simulink model "VB_RIFKF_GNSS_INS25"  (R2023a)
settings: Solver=FixedStepAuto  StartTime=0  StopTime=500  FixedStep=0.01  RelTol=1e-3
InitFcn:
  | resilient_initNavigation1216;
  | init_param;
undefined symbols (not defined in the file or in its folder): dt, g0, gam0_rad, ISUS_flag, magnitude, p, P0, P0_RIEKF, param, pd0, pe0, phi0_rad, pn0, psi, psi0_rad, state_dim, vd0, ve0, vn0
libraries: simulink_extras x68, dspstat3 x54, sharedtransform x47, simulink x43, matrix_library x9, sharedTrackingLibrary x5, dspfactors x4, aerolibconvert2 x3, aerolibtransform2 x3
(part 8 of 22)

== system VB_RIFKF_GNSS_INS25/ER EKF/Error State Kalman Filter/Extended Kalman Filter2 ==
  Q : Inport
  Enable1 : Inport  Port=2
  y1 : Inport  Port=3
  R1 : Inport  Port=4
  BlockOrdering : Constant  Value=true()  OutDataTypeStr=boolean
  Correct1 : Subsystem  AncestorBlock=sharedTrackingLibrary/Extras/EKFCorrect  TreatAsAtomicUnit=on  SystemSampleTime=p.SampleTimes.MeasurementFcn(1)  mask(EKFCorrect){ProcessedMaskData=p}
      mask init: same as VB_RIFKF_GNSS_INS25/ER EKF/Error State Kalman Filter/Extended Kalman Filter1/Correct1
      settings: LibrarySourceBlock=sharedTrackingLibrary/Extras/EKFCorrect
  DataStoreMemory - P : DataStoreMemory  DataStoreName=P  InitialValue=p.InitialCovariance  ShowAdditionalParam=off  OutDataTypeStr=p.DataType
  DataStoreMemory - x : DataStoreMemory  DataStoreName=x  InitialValue=p.InitialState  ShowAdditionalParam=off  OutDataTypeStr=p.DataType
  DataTypeConversion_Enable1 : DataTypeConversion  OutDataTypeStr=boolean  SaturateOnIntegerOverflow=off  RndMeth=Floor
  DataTypeConversion_Q : DataTypeConversion  OutDataTypeStr=p.DataType  SaturateOnIntegerOverflow=off  RndMeth=Floor
  DataTypeConversion_R1 : DataTypeConversion  OutDataTypeStr=p.DataType  SaturateOnIntegerOverflow=off  RndMeth=Floor
  DataTypeConversion_uMeas1 : DataTypeConversion  OutDataTypeStr=p.DataType  SaturateOnIntegerOverflow=off  RndMeth=Floor
  DataTypeConversion_uState : DataTypeConversion  OutDataTypeStr=p.DataType  SaturateOnIntegerOverflow=off  RndMeth=Floor
  DataTypeConversion_y1 : DataTypeConversion  OutDataTypeStr=p.DataType  SaturateOnIntegerOverflow=off  RndMeth=Floor
  MeasurementFcn1Inputs : Constant  Value=0  OutDataTypeStr=p.DataType  SampleTime=p.SampleTimes.MeasurementFcn(1)
  Output : Subsystem  TreatAsAtomicUnit=on  SystemSampleTime=p.SampleTimes.Output
  Predict : Subsystem  TreatAsAtomicUnit=on  SystemSampleTime=p.SampleTimes.StateTransitionFcn  mask(EKFPredict){ProcessedMaskData=p}
      mask init: same as VB_RIFKF_GNSS_INS25/ER EKF/Error State Kalman Filter/Extended Kalman Filter1/Predict
  StateTransitionFcnInputs : Constant  Value=0  OutDataTypeStr=p.DataType  SampleTime=p.SampleTimes.StateTransitionFcn
  checkMeasurementFcn1Signals : S-Function  FunctionName=ekfukfCheckSignals  Parameters=signalCheck.BlockPath, signalCheck.MeasurementFcn{1}.PortNames, signalCheck.MeasurementFcn{1}.SampleTime, signalCheck.DataType, signalCheck.MeasurementFcn{1}.PortDimensions, 1, signalCheck.MeasurementFcn{1}.HasAdditiveNoise  SFunctionDeploymentMode=off  EnableBusSupport=off
  checkStateTransitionFcnSignals : S-Function  FunctionName=ekfukfCheckSignals  Parameters=signalCheck.BlockPath, signalCheck.StateTransitionFcn.PortNames, signalCheck.StateTransitionFcn.SampleTime, signalCheck.DataType, signalCheck.StateTransitionFcn.PortDimensions, 0, signalCheck.StateTransitionFcn.HasAdditiveNoise  SFunctionDeploymentMode=off  EnableBusSupport=off
  xhat : Outport  VectorParamsAs1DForOutWhenUnconnected=off
  P : Outport  Port=2
  wires:
  y1/1 -> checkMeasurementFcn1Signals/2, DataTypeConversion_y1/1
  R1/1 -> checkMeasurementFcn1Signals/3, DataTypeConversion_R1/1
  Q/1 -> checkStateTransitionFcnSignals/1, DataTypeConversion_Q/1
  DataTypeConversion_Q/1 -> Predict/1(Q)
  Enable1/1 -> checkMeasurementFcn1Signals/1, DataTypeConversion_Enable1/1
  DataTypeConversion_Enable1/1 -> Correct1/Enable
  Output/2(P) -> P/1
  Output/1(x) -> xhat/1
  StateTransitionFcnInputs/1 -> checkStateTransitionFcnSignals/2, DataTypeConversion_uState/1
  DataTypeConversion_uState/1 -> Predict/2(uState)
  DataTypeConversion_y1/1 -> Correct1/1(yMeas)
  MeasurementFcn1Inputs/1 -> checkMeasurementFcn1Signals/4, DataTypeConversion_uMeas1/1
  DataTypeConversion_R1/1 -> Correct1/2(R)
  DataTypeConversion_uMeas1/1 -> Correct1/3(uMeas)
  BlockOrdering/1 -> [FirstOperation]
  [FirstOperation] -> Correct1/4(uBlockOrdering)
  [AfterCorrect] -> Output/1(uBlockOrdering)
  Output/3(yBlockOrdering) -> [AfterOutput]
  [AfterOutput] -> Predict/3(uBlockOrdering)
  Correct1/1(yBlockOrdering) -> [AfterCorrect]

== system VB_RIFKF_GNSS_INS25/ER EKF/Error State Kalman Filter/Simulink Function - GPS Measurements ==
  GPSMeasurementFcn : TriggerPort  TriggerType=function-call  IsSimulinkFunction=on  FunctionName=GPSMeasurementFcn  FunctionVisibility=scoped  VariantControl=Variant
  Add : Sum
  Constant6 : Constant  Value=[eye(6),zeros(6,9)]  OutDataTypeStr=single
  Product : Product  Multiplication=Matrix(*)
  x : ArgIn  DisableCoverage=on  OutDataTypeStr=single  PortDimensions=15  ArgumentName=x
  v : ArgIn  DisableCoverage=on  Port=2  OutDataTypeStr=single  PortDimensions=6  ArgumentName=v
  y : ArgOut  DisableCoverage=on  OutDataTypeStr=single  PortDimensions=6  ArgumentName=y
  wires:
  Add/1 -> y/1
  Product/1 -> Add/1
  x/1 -> Product/2
  Constant6/1 -> Product/1
  v/1 -> Add/2

== system VB_RIFKF_GNSS_INS25/ER EKF/Error State Kalman Filter/Simulink Function - GPS Measurements1 ==
  DCM_b_n : Inport
  DynamicMeasurementFcn_Dyn : TriggerPort  TriggerType=function-call  IsSimulinkFunction=on  FunctionName=DynamicMeasurementFcn_Dyn  FunctionVisibility=scoped  VariantControl=Variant
  Add : Sum  Commented=on
  Add1 : Sum
  Constant : Constant  Commented=on  Value=dt  OutDataTypeStr=single
  Constant6 : Constant  Value=[zeros(3,3),eye(3),zeros(3,12);zeros(3,15),eye(3)]  OutDataTypeStr=single
  Data Type Conversion6 : DataTypeConversion  Commented=on  OutDataTypeStr=single  SaturateOnIntegerOverflow=off  RndMeth=Floor
  From7 : From  Commented=on  GotoTag=DCM_b_n
  Goto : Goto  Commented=on  GotoTag=DCM_b_n
  MATLAB Function1 : MATLAB Function  Commented=on  TreatAsAtomicUnit=on
  Product : Product  Commented=on  Multiplication=Matrix(*)
  Product1 : Product  Multiplication=Matrix(*)
  x : ArgIn  DisableCoverage=on  OutDataTypeStr=single  PortDimensions=18  ArgumentName=x
  v : ArgIn  DisableCoverage=on  Port=2  OutDataTypeStr=single  PortDimensions=6  ArgumentName=v
  y : ArgOut  DisableCoverage=on  OutDataTypeStr=single  PortDimensions=6  ArgumentName=y
  wires:
  x/1 -> Product1/2
  Constant6/1 -> Product1/1
  Product1/1 -> Add1/1
  v/1 -> Add1/2
  Add1/1 -> y/1
  Data Type Conversion6/1 -> Product/1
  DCM_b_n/1 -> Goto/1
  Constant/1 -> MATLAB Function1/2(dt)
  From7/1 -> MATLAB Function1/1(Cbn)
  MATLAB Function1/1(H) -> Data Type Conversion6/1
  Product/1 -> Add/1

== system VB_RIFKF_GNSS_INS25/ER EKF/Error State Kalman Filter/Simulink Function - GPS Measurements2 ==
  ZUPTMeasurementFcn2 : TriggerPort  TriggerType=function-call  IsSimulinkFunction=on  FunctionName=ZUPTMeasurementFcn2  FunctionVisibility=scoped  VariantControl=Variant
  Add : Sum
  Constant6 : Constant  Value=[zeros(3,3),eye(3),zeros(3,12)]  OutDataTypeStr=single
  Product : Product  Multiplication=Matrix(*)
  x : ArgIn  DisableCoverage=on  OutDataTypeStr=single  PortDimensions=18  ArgumentName=x
  v : ArgIn  DisableCoverage=on  Port=2  OutDataTypeStr=single  PortDimensions=3  ArgumentName=v
  y : ArgOut  DisableCoverage=on  OutDataTypeStr=single  PortDimensions=3  ArgumentName=y
  wires:
  v/1 -> Add/2
  Constant6/1 -> Product/1
  x/1 -> Product/2
  Product/1 -> Add/1
  Add/1 -> y/1

== system VB_RIFKF_GNSS_INS25/ER EKF/Error State Kalman Filter/Simulink Function - State Transition ==
  DCM_b_n : Inport
  wxyz : Inport  Port=2
  fbxyz : Inport  Port=3
  stateTransitionFcn : TriggerPort  TriggerType=function-call  IsSimulinkFunction=on  FunctionName=stateTransitionFcn  FunctionVisibility=scoped  VariantControl=Variant
  Add : Sum
  Cal Phi : Subsystem
  Constant : Constant  Value=0.01  OutDataTypeStr=single
  Data Type Conversion1 : DataTypeConversion  OutDataTypeStr=single  SaturateOnIntegerOverflow=off  RndMeth=Floor
  Data Type Conversion6 : DataTypeConversion  OutDataTypeStr=single  SaturateOnIntegerOverflow=off  RndMeth=Floor
  MATLAB Function : MATLAB Function  TreatAsAtomicUnit=on
  Product1 : Product  Multiplication=Matrix(*)
  Product2 : Product  Multiplication=Matrix(*)
  Transpose : Math  Operator=transpose
  x : ArgIn  DisableCoverage=on  OutDataTypeStr=single  PortDimensions=15  ArgumentName=x
  w : ArgIn  Port=2  OutDataTypeStr=single  PortDimensions=12  ArgumentName=w
  xNext : ArgOut  DisableCoverage=on  OutDataTypeStr=single  PortDimensions=15  ArgumentName=xNext
  wires:
  Data Type Conversion6/1 -> Add/2
  Data Type Conversion1/1 -> Add/1
  Cal Phi/1(Phi) -> Product2/1
  fbxyz/1 -> [fbxyz]
  wxyz/1 -> [wxyz]
  DCM_b_n/1 -> [DCM_b_n]
  Constant/1 -> MATLAB Function/3(dt)
  [wxyz] -> MATLAB Function/2(wxyz)
  Transpose/1 -> MATLAB Function/1(Cnb)
  [DCM_b_n] -> Transpose/1
  [DCM_b_n] -> Cal Phi/1(<DCM_b_n>)
  [wxyz] -> Cal Phi/2(wxyz)
  [fbxyz] -> Cal Phi/3(axyz)
  Add/1 -> xNext/1
  Product1/1 -> Data Type Conversion1/1
  w/1 -> Product1/2
  MATLAB Function/1(G) -> Product1/1
  Product2/1 -> Data Type Conversion6/1
  x/1 -> Product2/2

== system VB_RIFKF_GNSS_INS25/ER EKF/Error State Kalman Filter/Simulink Function - State Transition Jacobian ==
  DCM_b_n : Inport
  wxyz : Inport  Port=2
  fbxyz : Inport  Port=3
  stateTransitionJacobianFcn : TriggerPort  TriggerType=function-call  IsSimulinkFunction=on  FunctionName=stateTransitionJacobianFcn  FunctionVisibility=scoped  VariantControl=Variant
  Cal Phi1 : Subsystem
  Constant : Constant  Value=0.01  OutDataTypeStr=single
  Data Type Conversion1 : DataTypeConversion  OutDataTypeStr=single  SaturateOnIntegerOverflow=off  RndMeth=Floor
  Data Type Conversion6 : DataTypeConversion  OutDataTypeStr=single  SaturateOnIntegerOverflow=off  RndMeth=Floor
  MATLAB Function : MATLAB Function  TreatAsAtomicUnit=on
  Terminator : Terminator
  Terminator1 : Terminator
  Transpose : Math  Operator=transpose
  x : ArgIn  DisableCoverage=on  OutDataTypeStr=single  PortDimensions=15  ArgumentName=x
  w : ArgIn  Port=2  OutDataTypeStr=single  PortDimensions=12  ArgumentName=w
  A : ArgOut  DisableCoverage=on  OutDataTypeStr=single  PortDimensions=[15 15]  ArgumentName=A
  G : ArgOut  Port=2  OutDataTypeStr=single  PortDimensions=[15 12]  ArgumentName=G
  wires:
  Data Type Conversion1/1 -> G/1
  Data Type Conversion6/1 -> A/1
  Constant/1 -> MATLAB Function/3(dt)
  Transpose/1 -> MATLAB Function/1(Cnb)
  [DCM_b_n] -> Transpose/1
  [wxyz] -> MATLAB Function/2(wxyz)
  [DCM_b_n] -> Cal Phi1/1(<DCM_b_n>)
  [fbxyz] -> Cal Phi1/3(axyz)
  [wxyz] -> Cal Phi1/2(wxyz)
  wxyz/1 -> [wxyz]
  fbxyz/1 -> [fbxyz]
  DCM_b_n/1 -> [DCM_b_n]
  Cal Phi1/1(Phi) -> Data Type Conversion6/1
  w/1 -> Terminator1/1
  x/1 -> Terminator/1
  MATLAB Function/1(G) -> Data Type Conversion1/1

== system VB_RIFKF_GNSS_INS25/ER EKF/Error State Kalman Filter/Subsystem ==
  data : Inport
  Detect Change : simulink/Logic and Bit Operations/Detect Change  vinit=0  InputProcessing=Columns as channels (frame based)  OutDataTypeStr=boolean
  Detect Change1 : simulink/Logic and Bit Operations/Detect Change  vinit=0  InputProcessing=Columns as channels (frame based)  OutDataTypeStr=boolean
  From Workspace2 : FromWorkspace  VariableName=[time(1:(end-1)),FCS1.data_hf_st.lat(1:(end-1))]
  From Workspace7 : FromWorkspace  Commented=on  VariableName=[All.t',All.vn]
  Selector : Selector  InputPortWidth=3  IndexOptions=Index vector (dialog)  Indices=[3]  OutputSizes=1
  Zero-Order Hold : ZeroOrderHold  SampleTime=0.2
  Zero-Order Hold1 : ZeroOrderHold  SampleTime=0.01
  flag : Outport
  wires:
  Zero-Order Hold/1 -> Selector/1
  data/1 -> Zero-Order Hold/1
  Selector/1 -> Zero-Order Hold1/1
  Detect Change1/1 -> flag/1
  Zero-Order Hold1/1 -> Detect Change/1
  From Workspace2/1 -> Detect Change1/1  "lat"

== system VB_RIFKF_GNSS_INS25/ER EKF/INS propogation/Init_PVQ ==
  QGC_sensor_reinit : Inport
  accl_B_m/s2_LPF : Inport  Port=2
  Magn_B_guess_LPF : Inport  Port=3
  pos_NED : Inport  Port=4
  vel_NED : Inport  Port=5
  Add : Sum
  Add1 : Sum
  Constant : Constant  Value=[0 0 0 1]  OutDataTypeStr=single
  Constant1 : Constant  OutDataTypeStr=uint8
  Constant2 : Constant  Value=[0;0;0]  OutDataTypeStr=single
  Constant3 : Constant  Value=[0;0;0]  OutDataTypeStr=single
  Constant4 : Constant  Value=[vn0;ve0;vd0]  OutDataTypeStr=single
  Constant5 : Constant  Value=[pn0;pe0;pd0]  OutDataTypeStr=single
  Detect Increase : simulink/Logic and Bit Operations/Detect Increase  vinit=0.0  OutDataTypeStr=boolean
  Horizontal_attitude : Subsystem  TreatAsAtomicUnit=on
  Horizontal_attitude2 : Subsystem  Commented=on  TreatAsAtomicUnit=on
  Memory : Memory
  Scope : Scope  NumInputPorts=2
  Scope1 : Scope
  Scope2 : Scope
  Subsystem : Subsystem
  Subsystem1 : Subsystem
  Switch{,1..3} (4 alike) : Switch  Criteria=u2 > Threshold  SaturateOnIntegerOverflow=off  InputSameDT=off
  quat_0 : Outport
  v0 : Outport  Port=2
  p0 : Outport  Port=3
  wires:
  Subsystem1/1(mean_data) -> Horizontal_attitude/2(Magn_mean_B_guess_LPF)
  Subsystem/1(mean_data) -> Horizontal_attitude/1(accl_mean_B_m/s_LPF)
  Memory/1 -> Switch1/3
  Constant/1 -> Switch/3
  Horizontal_attitude/1(quat_0) -> Switch/1
  Constant1/1 -> Switch1/1
  Switch1/1 -> Memory/1, Switch2/2, Switch3/2, Switch/2, Scope1/1
  accl_B_m/s2_LPF/1 -> Subsystem/1(data)
  QGC_sensor_reinit/1 -> Detect Increase/1, Scope/1
  Magn_B_guess_LPF/1 -> Subsystem1/1(data)
  Detect Increase/1 -> Horizontal_attitude/Enable, Switch1/2, Scope/2
  Constant2/1 -> Switch2/3
  Constant3/1 -> Switch3/3
  Switch2/1 -> v0/1
  Switch3/1 -> p0/1
  Add1/1 -> Switch3/1
  Switch/1 -> Scope2/1, quat_0/1
  Constant4/1 -> Add/2
  vel_NED/1 -> Add/1
  Add/1 -> Switch2/1
  pos_NED/1 -> Add1/1
  Constant5/1 -> Add1/2

== system VB_RIFKF_GNSS_INS25/ER EKF/INS propogation/accl bias compensation ==
  raw <accl_B_m/s2_LPF> : Inport
  dda : Inport  Port=2
  Add2 : Sum
  Data Type Conversion6 : DataTypeConversion  OutDataTypeStr=single  SaturateOnIntegerOverflow=off  RndMeth=Floor
  error compensation1 : Subsystem
  fb : Outport  PortDimensions=3
  da : Outport  Port=2  PortDimensions=3
  wires:
  error compensation1/1(da) -> da/1, Add2/2
  Add2/1 -> Data Type Conversion6/1
  Data Type Conversion6/1 -> fb/1
  raw <accl_B_m/s2_LPF>/1 -> Add2/1
  dda/1 -> error compensation1/1(dda)

== system VB_RIFKF_GNSS_INS25/ER EKF/INS propogation/att_update ==
  dtheta : Inport
  gyro : Inport  Port=2
  quat_0 : Inport  Port=3  PortDimensions=4
  init_flag : Inport  Port=4
  Bus Creator : BusCreator  Inputs=2
  Data Type Conversion1 : DataTypeConversion  OutDataTypeStr=single  SaturateOnIntegerOverflow=off  RndMeth=Floor
  Data Type Conversion2 : DataTypeConversion  OutDataTypeStr=single  SaturateOnIntegerOverflow=off  RndMeth=Floor
  Data Type Conversion3 : DataTypeConversion  OutDataTypeStr=double  SaturateOnIntegerOverflow=off  RndMeth=Floor
  Data Type Conversion4 : DataTypeConversion  OutDataTypeStr=double  SaturateOnIntegerOverflow=off  RndMeth=Floor
  Delay : Delay  DelayLength=1  InitialConditionSource=Input port  ExternalReset=Level hold
      settings: InputPortMap=u0,r5,p4
  Detect Increase : simulink/Logic and Bit Operations/Detect Increase  vinit=0.0  OutDataTypeStr=boolean
  Gain : Gain  Gain=dt  OutDataTypeStr=double
  Gain1 : Gain  Gain=-1
  JPLQuatMult : MATLAB Function  TreatAsAtomicUnit=on
  JPLQuatMult1 : MATLAB Function  TreatAsAtomicUnit=on
  JPLrv2q : MATLAB Function  TreatAsAtomicUnit=on
  JPLrv2q1 : MATLAB Function  TreatAsAtomicUnit=on
  MATLAB Function1 : MATLAB Function  TreatAsAtomicUnit=on
  Scope : Scope
  Transpose1 : Math  Operator=transpose  SignedPower=on
  att_update : Outport
  wires:
  JPLQuatMult/1(q_t) -> JPLQuatMult1/2(quatB)  "q_update"
  Detect Increase/1 -> Delay/2
  init_flag/1 -> Detect Increase/1
  Bus Creator/1 -> att_update/1
  Data Type Conversion2/1 -> Transpose1/1  "DCM_n_b"
  MATLAB Function1/1(Rot) -> Data Type Conversion2/1
  quat_0/1 -> Delay/3
  Delay/1 -> JPLQuatMult/2(quatB)
  Gain/1 -> JPLrv2q/1(rotVec)  "correctedDelAng"
  JPLrv2q/1(quaternion) -> JPLQuatMult/1(quatA)
  Data Type Conversion1/1 -> Bus Creator/1  "q_update"
  Data Type Conversion3/1 -> MATLAB Function1/1(q), Delay/1, Data Type Conversion1/1  "q_update"
  gyro/1 -> Gain/1
  Transpose1/1 -> Bus Creator/2  "DCM_b_n"
  Data Type Conversion4/1 -> JPLrv2q1/1(deltaTheta)  "q_update"
  JPLrv2q1/1(updateQuat) -> JPLQuatMult1/1(quatA)
  dtheta/1 -> Gain1/1
  Gain1/1 -> Scope/1, Data Type Conversion4/1
  JPLQuatMult1/1(q_t) -> Data Type Conversion3/1  "q_update"

== system VB_RIFKF_GNSS_INS25/ER EKF/INS propogation/gyro bias compensation ==
  raw <gyro_B_rad/s_LPF> : Inport
  ddg : Inport  Port=2
  Measuemrnt Enable Flag : Inport  Port=3
  Add1 : Sum
  Data Type Conversion4 : DataTypeConversion  OutDataTypeStr=single  SaturateOnIntegerOverflow=off  RndMeth=Floor
  Scope1 : Scope
  error compensation : Subsystem
  wb : Outport  PortDimensions=3
  dg : Outport  Port=2  PortDimensions=3
  wires:
  ddg/1 -> error compensation/1(ddg)
  Add1/1 -> Data Type Conversion4/1
  Measuemrnt Enable Flag/1 -> error compensation/2(Enable)
  error compensation/1(dg) -> dg/1, Scope1/1, Add1/2
  raw <gyro_B_rad/s_LPF>/1 -> Add1/1
  Data Type Conversion4/1 -> wb/1

== system VB_RIFKF_GNSS_INS25/ER EKF/INS propogation/vel_pos_update ==
  <DCM_b_n> : Inport
  Ab : Inport  Port=2
  v0 : Inport  Port=3
  p0 : Inport  Port=4
  QGC_init : Inport  Port=5
  dp : Inport  Port=6
  dv : Inport  Port=7
  Kinematic Equation : Subsystem
  QGC_init1 : InportShadow  Port=5
  pos update : Subsystem
  vel update : Subsystem
  p_k : Outport  PortDimensions=3
  V : Outport  Port=2  PortDimensions=3
  wires:
  <DCM_b_n>/1 -> Kinematic Equation/1(Cbn)
  Ab/1 -> Kinematic Equation/2(Ab)
  QGC_init/1 -> vel update/1(QGC_init)
  Kinematic Equation/1(An) -> vel update/2(An)
  dv/1 -> vel update/3(KFState_dv)
  v0/1 -> vel update/4(v0)
  dp/1 -> pos update/2(dp)
  p0/1 -> pos update/4(p0)
  pos update/1(p_k) -> p_k/1
  QGC_init1/1 -> pos update/3(QGC_init)
  vel update/1(vel_k) -> pos update/1(vel_k), V/1

== system VB_RIFKF_GNSS_INS25/ISUS_RIEKF1/Bus_Constructor2/Rotation_output ==
  RotationData : Inport
  Bus Creator : BusCreator  Inputs=4
  Bus Selector3 : BusSelector  OutputSignals=DCM_b_n
  Data Type Conversion1 : DataTypeConversion  OutDataTypeStr=single  SaturateOnIntegerOverflow=off  RndMeth=Floor
  Data Type Conversion11 : DataTypeConversion  OutDataTypeStr=single  SaturateOnIntegerOverflow=off  RndMeth=Floor
  Data Type Conversion12 : DataTypeConversion  OutDataTypeStr=double  SaturateOnIntegerOverflow=off  RndMeth=Floor
  Demux : Demux  Outputs=3
  Direction Cosine Matrix to Rotation Angles : sharedtransform/Direction Cosine Matrix to Rotation Angles  rotationOrder=ZYX  aMode=aMode  action=None  tolerance=eps(2)
      settings: LibrarySourceBlock=|
      | aerolibtransform2/Direction Cosine Matrix
      | to Rotation Angles
  Direction Cosine Matrix to Quaternions : sharedtransform/Direction Cosine Matrix  to Quaternions  aMode=0  action=None  tolerance=eps(2)
      settings: LibrarySourceBlock=|
      | aerolibtransform2/Direction Cosine Matrix
      | to Quaternions
  Radians to Degrees : simulink_extras/Transformations/Radians to Degrees
  Scope : Scope
  Signal Copy1 : SignalConversion  OverrideOpt=off
  Transpose : Math  Operator=transpose
  psi_theta_phi_rad : Outport
  wires:
  Direction Cosine Matrix to Quaternions/1 -> Data Type Conversion1/1  "q"
  Radians to Degrees/1 -> Data Type Conversion11/1
  Transpose/1 -> Data Type Conversion12/1
  Data Type Conversion12/1 -> Direction Cosine Matrix to Quaternions/1, Direction Cosine Matrix to Rotation Angles/1
  RotationData/1 -> Signal Copy1/1
  Signal Copy1/1 -> Bus Selector3/1
  Bus Selector3/1 -> Transpose/1  "<DCM_b_n>"
  Direction Cosine Matrix to Rotation Angles/1 -> Radians to Degrees/1
  Bus Creator/1 -> psi_theta_phi_rad/1
  Demux/1 -> Bus Creator/1  "psi_rad"
  Demux/2 -> Bus Creator/2  "theta_rad"
  Demux/3 -> Bus Creator/3, Scope/1  "phi_rad"
  Data Type Conversion11/1 -> Demux/1
  Data Type Conversion1/1 -> Bus Creator/4  "q"

== system VB_RIFKF_GNSS_INS25/ISUS_RIEKF1/Error State Kalman Filter M1/Cal Q1 ==
  Constant : Constant  Value=dt  OutDataTypeStr=double
  MATLAB Function1 : MATLAB Function  TreatAsAtomicUnit=on
  Qd : Outport
  wires:
  MATLAB Function1/1(Q) -> Qd/1
  Constant/1 -> MATLAB Function1/1(dt)

== system VB_RIFKF_GNSS_INS25/ISUS_RIEKF1/Error State Kalman Filter M1/Extended Kalman Filter M1 ==
  Q : Inport
  Enable1 : Inport  Port=2
  y1 : Inport  Port=3
  R1 : Inport  Port=4
  H : Inport  Port=5
  BlockOrdering : Constant  Value=true()  OutDataTypeStr=boolean
  Correct M1 : Subsystem  AncestorBlock=sharedTrackingLibrary/Extras/EKFCorrect  TreatAsAtomicUnit=on  SystemSampleTime=p.SampleTimes.MeasurementFcn(1)  mask(EKFCorrect){ProcessedMaskData=p}
      mask init: same as VB_RIFKF_GNSS_INS25/ER EKF/Error State Kalman Filter/Extended Kalman Filter1/Correct1
      settings: LibrarySourceBlock=sharedTrackingLibrary/Extras/EKFCorrect
  DataStoreMemory - P : DataStoreMemory  DataStoreName=P  InitialValue=p.InitialCovariance  ShowAdditionalParam=off  OutDataTypeStr=p.DataType
  DataStoreMemory - x : DataStoreMemory  DataStoreName=x  InitialValue=p.InitialState  ShowAdditionalParam=off  OutDataTypeStr=p.DataType
  DataTypeConversion_Enable1 : DataTypeConversion  OutDataTypeStr=boolean  SaturateOnIntegerOverflow=off  RndMeth=Floor
  DataTypeConversion_Q : DataTypeConversion  OutDataTypeStr=p.DataType  SaturateOnIntegerOverflow=off  RndMeth=Floor
  DataTypeConversion_R1 : DataTypeConversion  OutDataTypeStr=p.DataType  SaturateOnIntegerOverflow=off  RndMeth=Floor
  DataTypeConversion_uMeas1 : DataTypeConversion  OutDataTypeStr=p.DataType  SaturateOnIntegerOverflow=off  RndMeth=Floor
  DataTypeConversion_uState : DataTypeConversion  OutDataTypeStr=p.DataType  SaturateOnIntegerOverflow=off  RndMeth=Floor
  DataTypeConversion_y1 : DataTypeConversion  OutDataTypeStr=p.DataType  SaturateOnIntegerOverflow=off  RndMeth=Floor
  MeasurementFcn1Inputs : Constant  Value=0  OutDataTypeStr=p.DataType  SampleTime=p.SampleTimes.MeasurementFcn(1)
  Output : Subsystem  TreatAsAtomicUnit=on  SystemSampleTime=p.SampleTimes.Output
  Predict : Subsystem  TreatAsAtomicUnit=on  SystemSampleTime=p.SampleTimes.StateTransitionFcn  mask(EKFPredict){ProcessedMaskData=p}
      mask init: same as VB_RIFKF_GNSS_INS25/ER EKF/Error State Kalman Filter/Extended Kalman Filter1/Predict
  StateTransitionFcnInputs : Constant  Value=0  OutDataTypeStr=p.DataType  SampleTime=p.SampleTimes.StateTransitionFcn
  checkMeasurementFcn1Signals : S-Function  FunctionName=ekfukfCheckSignals  Parameters=signalCheck.BlockPath, signalCheck.MeasurementFcn{1}.PortNames, signalCheck.MeasurementFcn{1}.SampleTime, signalCheck.DataType, signalCheck.MeasurementFcn{1}.PortDimensions, 1, signalCheck.MeasurementFcn{1}.HasAdditiveNoise  SFunctionDeploymentMode=off  EnableBusSupport=off
  checkStateTransitionFcnSignals : S-Function  FunctionName=ekfukfCheckSignals  Parameters=signalCheck.BlockPath, signalCheck.StateTransitionFcn.PortNames, signalCheck.StateTransitionFcn.SampleTime, signalCheck.DataType, signalCheck.StateTransitionFcn.PortDimensions, 0, signalCheck.StateTransitionFcn.HasAdditiveNoise  SFunctionDeploymentMode=off  EnableBusSupport=off
  xhat : Outport  VectorParamsAs1DForOutWhenUnconnected=off
  P : Outport  Port=2
  wires:
  Output/2(P) -> P/1
  Correct M1/1(yBlockOrdering) -> [AfterCorrect]
  Output/1(x) -> xhat/1
  y1/1 -> checkMeasurementFcn1Signals/2, DataTypeConversion_y1/1
  R1/1 -> checkMeasurementFcn1Signals/3, DataTypeConversion_R1/1
  Q/1 -> checkStateTransitionFcnSignals/1, DataTypeConversion_Q/1
  DataTypeConversion_Q/1 -> Predict/1(Q)
  Enable1/1 -> checkMeasurementFcn1Signals/1, DataTypeConversion_Enable1/1
  DataTypeConversion_Enable1/1 -> Correct M1/Enable
  StateTransitionFcnInputs/1 -> checkStateTransitionFcnSignals/2, DataTypeConversion_uState/1
  DataTypeConversion_uState/1 -> Predict/2(uState)
  DataTypeConversion_y1/1 -> Correct M1/1(yMeas)
  MeasurementFcn1Inputs/1 -> checkMeasurementFcn1Signals/4, DataTypeConversion_uMeas1/1
  DataTypeConversion_R1/1 -> Correct M1/2(R)
  DataTypeConversion_uMeas1/1 -> Correct M1/3(uMeas)
  BlockOrdering/1 -> [FirstOperation]
  [FirstOperation] -> Correct M1/4(uBlockOrdering)
  [AfterCorrect] -> Output/1(uBlockOrdering)
  Output/3(yBlockOrdering) -> [AfterOutput]
  [AfterOutput] -> Predict/3(uBlockOrdering)
  H/1 -> Correct M1/5(H)

== system VB_RIFKF_GNSS_INS25/ISUS_RIEKF1/Error State Kalman Filter M1/Extended Kalman Filter M2 ==
  Q : Inport
  Enable1 : Inport  Port=2
  y1 : Inport  Port=3
  R1 : Inport  Port=4
  BlockOrdering : Constant  Value=true()  OutDataTypeStr=boolean
  Correct M1 : Subsystem  AncestorBlock=sharedTrackingLibrary/Extras/EKFCorrect  TreatAsAtomicUnit=on  SystemSampleTime=p.SampleTimes.MeasurementFcn(1)  mask(EKFCorrect){ProcessedMaskData=p}
      mask init: same as VB_RIFKF_GNSS_INS25/ER EKF/Error State Kalman Filter/Extended Kalman Filter1/Correct1
      settings: LibrarySourceBlock=sharedTrackingLibrary/Extras/EKFCorrect
  DataStoreMemory - P : DataStoreMemory  DataStoreName=P  InitialValue=p.InitialCovariance  ShowAdditionalParam=off  OutDataTypeStr=p.DataType
  DataStoreMemory - x : DataStoreMemory  DataStoreName=x  InitialValue=p.InitialState  ShowAdditionalParam=off  OutDataTypeStr=p.DataType
  DataTypeConversion_Enable1 : DataTypeConversion  OutDataTypeStr=boolean  SaturateOnIntegerOverflow=off  RndMeth=Floor
  DataTypeConversion_Q : DataTypeConversion  OutDataTypeStr=p.DataType  SaturateOnIntegerOverflow=off  RndMeth=Floor
  DataTypeConversion_R1 : DataTypeConversion  OutDataTypeStr=p.DataType  SaturateOnIntegerOverflow=off  RndMeth=Floor
  DataTypeConversion_uMeas1 : DataTypeConversion  OutDataTypeStr=p.DataType  SaturateOnIntegerOverflow=off  RndMeth=Floor
  DataTypeConversion_uState : DataTypeConversion  OutDataTypeStr=p.DataType  SaturateOnIntegerOverflow=off  RndMeth=Floor
  DataTypeConversion_y1 : DataTypeConversion  OutDataTypeStr=p.DataType  SaturateOnIntegerOverflow=off  RndMeth=Floor
  MeasurementFcn1Inputs : Constant  Value=0  OutDataTypeStr=p.DataType  SampleTime=p.SampleTimes.MeasurementFcn(1)
  Output : Subsystem  TreatAsAtomicUnit=on  SystemSampleTime=p.SampleTimes.Output
  Predict : Subsystem  TreatAsAtomicUnit=on  SystemSampleTime=p.SampleTimes.StateTransitionFcn  mask(EKFPredict){ProcessedMaskData=p}
      mask init: same as VB_RIFKF_GNSS_INS25/ER EKF/Error State Kalman Filter/Extended Kalman Filter1/Predict
  StateTransitionFcnInputs : Constant  Value=0  OutDataTypeStr=p.DataType  SampleTime=p.SampleTimes.StateTransitionFcn
  checkMeasurementFcn1Signals : S-Function  FunctionName=ekfukfCheckSignals  Parameters=signalCheck.BlockPath, signalCheck.MeasurementFcn{1}.PortNames, signalCheck.MeasurementFcn{1}.SampleTime, signalCheck.DataType, signalCheck.MeasurementFcn{1}.PortDimensions, 1, signalCheck.MeasurementFcn{1}.HasAdditiveNoise  SFunctionDeploymentMode=off  EnableBusSupport=off
  checkStateTransitionFcnSignals : S-Function  FunctionName=ekfukfCheckSignals  Parameters=signalCheck.BlockPath, signalCheck.StateTransitionFcn.PortNames, signalCheck.StateTransitionFcn.SampleTime, signalCheck.DataType, signalCheck.StateTransitionFcn.PortDimensions, 0, signalCheck.StateTransitionFcn.HasAdditiveNoise  SFunctionDeploymentMode=off  EnableBusSupport=off
  xhat : Outport  VectorParamsAs1DForOutWhenUnconnected=off
  P : Outport  Port=2
  wires:
  [AfterOutput] -> Predict/3(uBlockOrdering)
  Output/3(yBlockOrdering) -> [AfterOutput]
  [AfterCorrect] -> Output/1(uBlockOrdering)
  [FirstOperation] -> Correct M1/4(uBlockOrdering)
  BlockOrdering/1 -> [FirstOperation]
  DataTypeConversion_uMeas1/1 -> Correct M1/3(uMeas)
  DataTypeConversion_R1/1 -> Correct M1/2(R)
  MeasurementFcn1Inputs/1 -> DataTypeConversion_uMeas1/1, checkMeasurementFcn1Signals/4
  DataTypeConversion_y1/1 -> Correct M1/1(yMeas)
  DataTypeConversion_uState/1 -> Predict/2(uState)
  StateTransitionFcnInputs/1 -> DataTypeConversion_uState/1, checkStateTransitionFcnSignals/2
  DataTypeConversion_Enable1/1 -> Correct M1/Enable
  Enable1/1 -> DataTypeConversion_Enable1/1, checkMeasurementFcn1Signals/1
  DataTypeConversion_Q/1 -> Predict/1(Q)
  Q/1 -> DataTypeConversion_Q/1, checkStateTransitionFcnSignals/1
  R1/1 -> DataTypeConversion_R1/1, checkMeasurementFcn1Signals/3
  y1/1 -> DataTypeConversion_y1/1, checkMeasurementFcn1Signals/2
  Output/1(x) -> xhat/1
  Correct M1/1(yBlockOrdering) -> [AfterCorrect]
  Output/2(P) -> P/1

== system VB_RIFKF_GNSS_INS25/ISUS_RIEKF1/Error State Kalman Filter M1/Simulink Function - GPS Measurements ==
  Rbn : Inport
  vn : Inport  Port=2
  pn : Inport  Port=3
  GPSMeasurementFcn_RIEKF : TriggerPort  TriggerType=function-call  IsSimulinkFunction=on  FunctionName=GPSMeasurementFcn_RIEKF  FunctionVisibility=scoped  VariantControl=Variant
  Add : Sum
  Data Type Conversion1 : DataTypeConversion  OutDataTypeStr=single  SaturateOnIntegerOverflow=off  RndMeth=Floor
  MATLAB Function : MATLAB Function  TreatAsAtomicUnit=on
  MATLAB Function1 : MATLAB Function  Commented=on  TreatAsAtomicUnit=on
  Product : Product  Multiplication=Matrix(*)
  pn1 : InportShadow  Port=3
  vn1 : InportShadow  Port=2
  x : ArgIn  DisableCoverage=on  OutDataTypeStr=single  PortDimensions=state_dim  ArgumentName=x
  v : ArgIn  DisableCoverage=on  Port=2  OutDataTypeStr=single  PortDimensions=6  ArgumentName=v
  y : ArgOut  DisableCoverage=on  OutDataTypeStr=single  PortDimensions=6  ArgumentName=y
  H : Outport
  wires:
  Data Type Conversion1/1 -> Product/1, H/1
  pn/1 -> MATLAB Function/2(pn)
  v/1 -> Add/2
  x/1 -> Product/2
  pn1/1 -> MATLAB Function1/3(pn)
  vn1/1 -> MATLAB Function1/2(vn)
  Rbn/1 -> MATLAB Function1/1(Rbn)
  vn/1 -> MATLAB Function/1(vn)
  Add/1 -> y/1
  Product/1 -> Add/1
  MATLAB Function/1(H) -> Data Type Conversion1/1

== system VB_RIFKF_GNSS_INS25/ISUS_RIEKF1/Error State Kalman Filter M1/Simulink Function - GPS Measurements1 ==
  vn : Inport
  pn : Inport  Port=2
  BaroMeasurementFcn_RIEKF : TriggerPort  TriggerType=function-call  IsSimulinkFunction=on  FunctionName=BaroMeasurementFcn_RIEKF  VariantControl=Variant
  Add : Sum
  Data Type Conversion1 : DataTypeConversion  OutDataTypeStr=single  SaturateOnIntegerOverflow=off  RndMeth=Floor
  MATLAB Function : MATLAB Function  TreatAsAtomicUnit=on
  Product : Product  Multiplication=Matrix(*)
  x : ArgIn  DisableCoverage=on  OutDataTypeStr=single  PortDimensions=state_dim  ArgumentName=x
  v : ArgIn  DisableCoverage=on  Port=2  OutDataTypeStr=single  ArgumentName=v
  y : ArgOut  DisableCoverage=on  OutDataTypeStr=single  ArgumentName=y
  wires:
  Data Type Conversion1/1 -> Product/1
  pn/1 -> MATLAB Function/2(pn)
  v/1 -> Add/2
  x/1 -> Product/2
  vn/1 -> MATLAB Function/1(vn)
  Add/1 -> y/1
  Product/1 -> Add/1
  MATLAB Function/1(H_baro) -> Data Type Conversion1/1

== system VB_RIFKF_GNSS_INS25/ISUS_RIEKF1/Error State Kalman Filter M1/Simulink Function - GPS Measurements2 ==
  Rbn : Inport
  Magn : Inport  Port=2
  xstate : Inport  Port=3
  MagnMeasurementFcn_RIEKF : TriggerPort  TriggerType=function-call  IsSimulinkFunction=on  FunctionName=MagnMeasurementFcn_RIEKF  VariantControl=Variant
  Add : Sum
  Data Type Conversion1 : DataTypeConversion  OutDataTypeStr=single  SaturateOnIntegerOverflow=off  RndMeth=Floor
  MATLAB Function : MATLAB Function  TreatAsAtomicUnit=on
  Product : Product  Multiplication=Matrix(*)
  Selector : Selector  InputPortWidth=state_dim  IndexOptions=Index vector (dialog)  Indices=[1 2 3]  OutputSizes=1
  x : ArgIn  DisableCoverage=on  OutDataTypeStr=single  PortDimensions=state_dim  ArgumentName=x
  v : ArgIn  DisableCoverage=on  Port=2  OutDataTypeStr=single  PortDimensions=3  ArgumentName=v
  y : ArgOut  DisableCoverage=on  OutDataTypeStr=single  PortDimensions=3  ArgumentName=y
  wires:
  Selector/1 -> MATLAB Function/3(dtheta)
  xstate/1 -> Selector/1
  Rbn/1 -> MATLAB Function/1(Rbn)
  Data Type Conversion1/1 -> Product/1
  v/1 -> Add/2
  x/1 -> Product/2
  Magn/1 -> MATLAB Function/2(Magn)
  Add/1 -> y/1
  Product/1 -> Add/1
  MATLAB Function/1(H) -> Data Type Conversion1/1

== system VB_RIFKF_GNSS_INS25/ISUS_RIEKF1/Error State Kalman Filter M1/Simulink Function - GPS Measurements3 ==
  Rbn : Inport
  vn : Inport  Port=2
  Rab : Inport  Port=3
  vel_wind_NED : Inport  Port=4
  AirspeedMeasurementFcn_RIEKF : TriggerPort  TriggerType=function-call  IsSimulinkFunction=on  FunctionName=AirspeedMeasurementFcn_RIEKF  VariantControl=Variant
  Add : Sum
  Data Type Conversion1 : DataTypeConversion  OutDataTypeStr=single  SaturateOnIntegerOverflow=off  RndMeth=Floor
  MATLAB Function : MATLAB Function  TreatAsAtomicUnit=on
  Product : Product  Multiplication=Matrix(*)
  x : ArgIn  DisableCoverage=on  OutDataTypeStr=single  PortDimensions=state_dim  ArgumentName=x
  v : ArgIn  DisableCoverage=on  Port=2  OutDataTypeStr=single  PortDimensions=3  ArgumentName=v
  y : ArgOut  DisableCoverage=on  OutDataTypeStr=single  PortDimensions=3  ArgumentName=y
  wires:
  vel_wind_NED/1 -> MATLAB Function/4(v_wind)
  Rab/1 -> MATLAB Function/2(Rab)
  vn/1 -> MATLAB Function/3(vn)
  Rbn/1 -> MATLAB Function/1(Rbn)
  Data Type Conversion1/1 -> Product/1
  v/1 -> Add/2
  x/1 -> Product/2
  Add/1 -> y/1
  Product/1 -> Add/1
  MATLAB Function/1(H) -> Data Type Conversion1/1

== system VB_RIFKF_GNSS_INS25/ISUS_RIEKF1/Error State Kalman Filter M1/Simulink Function - State Transition ==
  DCM_b_n : Inport
  vn : Inport  Port=2  PortDimensions=[3,1]
  pn : Inport  Port=3  PortDimensions=[3,1]
  stateTransitionFcn_RIEKF : TriggerPort  TriggerType=function-call  IsSimulinkFunction=on  FunctionName=stateTransitionFcn_RIEKF  FunctionVisibility=scoped  VariantControl=Variant
  Add : Sum
  Cal Phi : Subsystem
  Constant : Constant  Value=dt  OutDataTypeStr=single
  Data Type Conversion1 : DataTypeConversion  OutDataTypeStr=single  SaturateOnIntegerOverflow=off  RndMeth=Floor
  Data Type Conversion6 : DataTypeConversion  OutDataTypeStr=single  SaturateOnIntegerOverflow=off  RndMeth=Floor
  MATLAB Function : MATLAB Function  TreatAsAtomicUnit=on
  Product1 : Product  Multiplication=Matrix(*)
  Product2 : Product  Multiplication=Matrix(*)
  x : ArgIn  DisableCoverage=on  OutDataTypeStr=single  PortDimensions=state_dim  ArgumentName=x
  w : ArgIn  Port=2  OutDataTypeStr=single  PortDimensions=cov_dim  ArgumentName=w
  xNext : ArgOut  DisableCoverage=on  OutDataTypeStr=single  PortDimensions=state_dim  ArgumentName=xNext
  wires:
  Data Type Conversion1/1 -> Add/1
  pn/1 -> Cal Phi/3(pn), MATLAB Function/3(pn)
  vn/1 -> Cal Phi/2(vn), MATLAB Function/2(vn)
  [DCM_b_n] -> Cal Phi/1(Rbn)
  Data Type Conversion6/1 -> Add/2
  Cal Phi/1(Phi) -> Product2/1
  DCM_b_n/1 -> [DCM_b_n]
  Constant/1 -> MATLAB Function/4(dt)
  [DCM_b_n] -> MATLAB Function/1(Rbn)
  Add/1 -> xNext/1
  Product1/1 -> Data Type Conversion1/1
  w/1 -> Product1/2
  MATLAB Function/1(G) -> Product1/1
  Product2/1 -> Data Type Conversion6/1
  x/1 -> Product2/2

== system VB_RIFKF_GNSS_INS25/ISUS_RIEKF1/Error State Kalman Filter M1/Simulink Function - State Transition1 ==
  DCM_b_n : Inport
  vn : Inport  Port=2  PortDimensions=[3,1]
  pn : Inport  Port=3  PortDimensions=[3,1]
  stateFcn_RIEKFJacobian : TriggerPort  TriggerType=function-call  IsSimulinkFunction=on  FunctionName=stateFcn_RIEKFJacobian  FunctionVisibility=scoped  VariantControl=Variant
  Cal Phi : Subsystem
  Constant : Constant  Value=dt  OutDataTypeStr=single
  Data Type Conversion1 : DataTypeConversion  OutDataTypeStr=single  SaturateOnIntegerOverflow=off  RndMeth=Floor
  Data Type Conversion6 : DataTypeConversion  OutDataTypeStr=single  SaturateOnIntegerOverflow=off  RndMeth=Floor
  MATLAB Function : MATLAB Function  TreatAsAtomicUnit=on
  Terminator : Terminator
  Terminator1 : Terminator
  x : ArgIn  DisableCoverage=on  OutDataTypeStr=single  PortDimensions=state_dim  ArgumentName=x
  w : ArgIn  Port=2  OutDataTypeStr=single  PortDimensions=cov_dim  ArgumentName=w
  A : ArgOut  DisableCoverage=on  OutDataTypeStr=single  PortDimensions=[state_dim,state_dim]  ArgumentName=A
  G : ArgOut  Port=2  OutDataTypeStr=single  PortDimensions=[15,12]  ArgumentName=G
  wires:
  Data Type Conversion1/1 -> A/1
  Data Type Conversion6/1 -> G/1
  Cal Phi/1(Phi) -> Data Type Conversion1/1
  MATLAB Function/1(G) -> Data Type Conversion6/1
  x/1 -> Terminator1/1
  w/1 -> Terminator/1
  [DCM_b_n] -> MATLAB Function/1(Rbn)
  Constant/1 -> MATLAB Function/4(dt)
  DCM_b_n/1 -> [DCM_b_n]
  [DCM_b_n] -> Cal Phi/1(Rbn)
  vn/1 -> MATLAB Function/2(vn), Cal Phi/2(vn)
  pn/1 -> MATLAB Function/3(pn), Cal Phi/3(pn)

== system VB_RIFKF_GNSS_INS25/ISUS_RIEKF1/Error State Kalman Filter M1/Subsystem ==
  data : Inport
  Detect Change : simulink/Logic and Bit Operations/Detect Change  vinit=0  InputProcessing=Columns as channels (frame based)  OutDataTypeStr=boolean
  Selector : Selector  InputPortWidth=3  IndexOptions=Index vector (dialog)  Indices=[3]  OutputSizes=1
  Zero-Order Hold : ZeroOrderHold  SampleTime=0.2
  Zero-Order Hold1 : ZeroOrderHold  SampleTime=0.01
  flag : Outport
  wires:
  Zero-Order Hold/1 -> Selector/1
  data/1 -> Zero-Order Hold/1
  Selector/1 -> Zero-Order Hold1/1
  Detect Change/1 -> flag/1
  Zero-Order Hold1/1 -> Detect Change/1

== system VB_RIFKF_GNSS_INS25/ISUS_RIEKF1/Error State Kalman Filter M1/Subsystem1 ==
  v_I : Inport
  v_G : Inport  Port=2
  p_I : Inport  Port=3
  p_G : Inport  Port=4
  Add1 : Sum  Inputs=+-
  Add2 : Sum  Inputs=+-
  Data Type Conversion : DataTypeConversion  OutDataTypeStr=single  SaturateOnIntegerOverflow=off  RndMeth=Floor
  Data Type Conversion2 : DataTypeConversion  OutDataTypeStr=single  SaturateOnIntegerOverflow=off  RndMeth=Floor
  Gain : Gain  Gain=-1
  Mux2 : Mux  Inputs=2
  dv/dp : Outport
  wires:
  p_G/1 -> Add1/2
  Gain/1 -> dv/dp/1
  v_I/1 -> Add2/1
  Add2/1 -> Data Type Conversion2/1
  Add1/1 -> Data Type Conversion/1
  p_I/1 -> Add1/1
  Data Type Conversion/1 -> Mux2/2
  v_G/1 -> Add2/2
  Data Type Conversion2/1 -> Mux2/1
  Mux2/1 -> Gain/1

== system VB_RIFKF_GNSS_INS25/ISUS_RIEKF1/Error State Kalman Filter M1/Subsystem3 ==
  data : Inport
  Constant : Constant  Value=false
  Detect Change : simulink/Logic and Bit Operations/Detect Change  vinit=0  InputProcessing=Columns as channels (frame based)  OutDataTypeStr=boolean
  Digital Clock : DigitalClock  SampleTime=0.01
  From Workspace1 : FromWorkspace  Commented=on  VariableName=[All.t',All.vn]
  From Workspace2 : FromWorkspace  VariableName=[time(1:(end-1)),FCS1.data_hf_st.lat(1:(end-1))]
  Selector : Selector  InputPortWidth=3  IndexOptions=Index vector (dialog)  Indices=[3]  OutputSizes=1
  Switch : Switch  Criteria=u2 > Threshold  Threshold=1  SaturateOnIntegerOverflow=off  InputSameDT=off
  flag : Outport
  wires:
  Detect Change/1 -> Switch/1
  Digital Clock/1 -> Switch/2
  Constant/1 -> Switch/3
  From Workspace2/1 -> Detect Change/1  "lat"
  data/1 -> Selector/1
  Switch/1 -> flag/1

== system VB_RIFKF_GNSS_INS25/ISUS_RIEKF1/Error State Kalman Filter M1/bak ==
  From1 : From  Commented=on  GotoTag=wxyz
  From11 : From  Commented=on  GotoTag=p_INS
  From14 : From  Commented=on  GotoTag=DCM_b_n
  From2 : From  Commented=on  GotoTag=fbxyz
  From3 : From  Commented=on  GotoTag=ZUPTenable
  From4 : From  Commented=on  GotoTag=v_INS
  From5 : From  Commented=on  GotoTag=fex
  From6 : From  Commented=on  GotoTag=DCM_b_n
  From9 : From  Commented=on  GotoTag=DCM_b_n
  Goto6 : Goto  Commented=on  GotoTag=ZUPTenable
  MATLAB Function1 : MATLAB Function  Commented=on  TreatAsAtomicUnit=on
  Memory1 : Memory  Commented=on
  RIEKF : MATLAB Function  Commented=on  TreatAsAtomicUnit=on
  Rate Transition2 : RateTransition  Commented=on  OutPortSampleTime=dt
  Scope10 : Scope  Commented=on  NumInputPorts=2
  Simulink Function - GPS Measurements1 : Subsystem  Commented=on  TreatAsAtomicUnit=on
  Simulink Function - GPS Measurements2 : Subsystem  Commented=on  TreatAsAtomicUnit=on
  Simulink Function - State Transition Jacobian : Subsystem  Commented=on  TreatAsAtomicUnit=on
  Unscented Kalman Filter1 : sharedTrackingLibrary/Unscented Kalman Filter  Commented=on  StateTransitionFcn=stateTransitionFcn_Dyn  HasAdditiveProcessNoise=Nonadditive  ProcessNoise=1  HasTimeVaryingProcessNoise=on  HasStateTransitionFcnExtraArgument=0  InitialState=zeros(18,1)  InitialStateCovariance=diag([1*ones(3,1);0.1*ones(3,1);0.001*ones(3,1);0.001*ones(6,1);0.1*ones(3,1)]);  Alpha=1e-2  Beta=2  Kappa=0  MeasurementFcn1=GPSMeasurementFcn_Dyn  HasMeasurementEnablePort1=on  HasAdditiveMeasurementNoise1=Nonadditive  MeasurementNoise1=1  HasTimeVaryingMeasurementNoise1=on  HasMeasurementFcnExtraArgument1=0  HasMeasurementWrapping1=off  MeasurementFcn2=DynamicMeasurementFcn_Dyn  HasMeasurementEnablePort2=on  HasAdditiveMeasurementNoise2=Nonadditive  MeasurementNoise2=1  HasTimeVaryingMeasurementNoise2=on  HasMeasurementFcnExtraArgument2=0  HasMeasurementWrapping2=off  MeasurementFcn3=myMeasurementFcn  HasMeasurementEnablePort3=off  HasAdditiveMeasurementNoise3=Additive  MeasurementNoise3=1  HasTimeVaryingMeasurementNoise3=off  HasMeasurementFcnExtraArgument3=0  HasMeasurementWrapping3=off  MeasurementFcn4=myMeasurementFcn  HasMeasurementEnablePort4=off  HasAdditiveMeasurementNoise4=Additive  MeasurementNoise4=1  HasTimeVaryingMeasurementNoise4=off  HasMeasurementFcnExtraArgument4=0  HasMeasurementWrapping4=off  MeasurementFcn5=myMeasurementFcn  HasMeasurementEnablePort5=off  HasAdditiveMeasurementNoise5=Additive  MeasurementNoise5=1  HasTimeVaryingMeasurementNoise5=off  HasMeasurementFcnExtraArgument5=0  HasMeasurementWrapping5=off  EnableMultirate=off  StateTransitionFcnSampleTime=1  MeasurementFcn1SampleTime=1  MeasurementFcn2SampleTime=1  MeasurementFcn3SampleTime=1  MeasurementFcn4SampleTime=1  MeasurementFcn5SampleTime=1  UseCurrentEstimator=on  OutputStateCovariance=on  DataType=single  SampleTime=0.01  NumberOfMeasurements=2
  Out1 : Outport
  wires:
  From14/1 -> Simulink Function - GPS Measurements1/1(DCM_b_n)
  From4/1 -> Simulink Function - State Transition Jacobian/2(vn)
  From9/1 -> Simulink Function - State Transition Jacobian/1(DCM_b_n)
  From11/1 -> Simulink Function - State Transition Jacobian/3(pn)
  From3/1 -> Rate Transition2/1
  MATLAB Function1/2(ZeroVelDetectFlagold) -> Scope10/2
  From6/1 -> MATLAB Function1/1(Cbn)
  From2/1 -> MATLAB Function1/3(fbxyz)
  From5/1 -> Memory1/1
  MATLAB Function1/1(ZeroVelDetectFlag) -> Goto6/1, Scope10/1
  From1/1 -> MATLAB Function1/2(wxyz)
  Rate Transition2/1 -> Out1/1
  Memory1/1 -> MATLAB Function1/4(fex)

== system VB_RIFKF_GNSS_INS25/ISUS_RIEKF1/INS propogation/Init_PVQ ==
  QGC_sensor_reinit : Inport
  accl_B_m/s2_LPF : Inport  Port=2
  Magn_B_guess_LPF : Inport  Port=3
  pos_NED : Inport  Port=4
  vel_NED : Inport  Port=5
  Add : Sum
  Add1 : Sum
  Constant1 : Constant  OutDataTypeStr=uint8
  Constant2 : Constant  Value=[0;0;0]  OutDataTypeStr=single
  Constant3 : Constant  Value=[0;0;0]  OutDataTypeStr=single
  Constant4 : Constant  Value=[vn0;ve0;vd0]  OutDataTypeStr=single
  Constant5 : Constant  Value=[pn0;pe0;pd0]  OutDataTypeStr=single
  Detect Increase : simulink/Logic and Bit Operations/Detect Increase  vinit=0.0  OutDataTypeStr=boolean
  Horizontal_attitude : Subsystem  TreatAsAtomicUnit=on
  Memory : Memory
  Scope : Scope  NumInputPorts=2
  Scope1 : Scope
  Subsystem : Subsystem
  Subsystem1 : Subsystem
  Subsystem2 : Subsystem
  Switch{,1..3} (4 alike) : Switch  Criteria=u2 > Threshold  SaturateOnIntegerOverflow=off  InputSameDT=off
  quat_0 : Outport
  v0 : Outport  Port=2
  p0 : Outport  Port=3
  wires:
  pos_NED/1 -> Add1/1
  Constant5/1 -> Add1/2
  Constant4/1 -> Add/2
  vel_NED/1 -> Add/1
  Switch/1 -> quat_0/1
  Subsystem1/1(mean_data) -> Horizontal_attitude/2(Magn_mean_B_guess_LPF)
  Subsystem/1(mean_data) -> Horizontal_attitude/1(accl_mean_B_m/s_LPF)
  Memory/1 -> Switch1/3
  Subsystem2/1(Quat0) -> Switch/3
  Horizontal_attitude/1(quat_0) -> Switch/1
  Constant1/1 -> Switch1/1
  Switch1/1 -> Memory/1, Switch2/2, Switch3/2, Switch/2, Scope1/1
  accl_B_m/s2_LPF/1 -> Subsystem/1(data)
  QGC_sensor_reinit/1 -> Detect Increase/1, Scope/1
  Magn_B_guess_LPF/1 -> Subsystem1/1(data)
  Detect Increase/1 -> Horizontal_attitude/Enable, Switch1/2, Scope/2
  Constant2/1 -> Switch2/3
  Constant3/1 -> Switch3/3
  Switch2/1 -> v0/1
  Switch3/1 -> p0/1
  Add1/1 -> Switch3/1
  Add/1 -> Switch2/1

== system VB_RIFKF_GNSS_INS25/ISUS_RIEKF1/INS propogation/accl bias compensation ==
  QGC_init : Inport
  raw <accl_B_m/s2_LPF> : Inport  Port=2
  dda : Inport  Port=3
  Add2 : Sum
  Data Type Conversion6 : DataTypeConversion  OutDataTypeStr=single  SaturateOnIntegerOverflow=off  RndMeth=Floor
  error compensation1 : Subsystem
  fb : Outport  PortDimensions=3
  da : Outport  Port=2  PortDimensions=3
  wires:
  QGC_init/1 -> error compensation1/2(QGC_init)
  error compensation1/1(da) -> da/1, Add2/2
  Add2/1 -> Data Type Conversion6/1
  Data Type Conversion6/1 -> fb/1
  raw <accl_B_m/s2_LPF>/1 -> Add2/1
  dda/1 -> error compensation1/1(dda)

== system VB_RIFKF_GNSS_INS25/ISUS_RIEKF1/INS propogation/att update ==
  dtheta : Inport
  gyro : Inport  Port=2
  quat_0 : Inport  Port=3  PortDimensions=4
  init_flag : Inport  Port=4
  Bus Creator1 : BusCreator  Inputs=1
  Constant : Constant  Value=dt
  Delay1 : Delay  DelayLength=1  InitialConditionSource=Input port  InitialCondition=0  ExternalReset=Level hold
      settings: InputPortMap=u0,r5,p4
  Detect Increase : simulink/Logic and Bit Operations/Detect Increase  vinit=0.0  OutDataTypeStr=boolean
  MATLAB Function : MATLAB Function  TreatAsAtomicUnit=on
  MATLAB Function2 : MATLAB Function  TreatAsAtomicUnit=on
  Quaternions to Direction Cosine Matrix : sharedtransform/Quaternions to  Direction Cosine Matrix  aMode=aMode
      settings: LibrarySourceBlock=|
      | aerolibtransform2/Quaternions to
      | Direction Cosine Matrix
  Scope : Scope
  Transpose : Math  Operator=transpose
  att_update1 : Outport
  wires:
  dtheta/1 -> Scope/1, MATLAB Function2/1(delta)
  MATLAB Function2/1(Rbn_correct) -> Bus Creator1/1  "DCM_b_n"
  MATLAB Function/1(Rbn) -> MATLAB Function2/2(Rbn)  "DCM_b_n"
  Bus Creator1/1 -> att_update1/1, Delay1/1
  Detect Increase/1 -> Delay1/2
  Delay1/1 -> MATLAB Function/1(Rbn_k_1)
  Transpose/1 -> Delay1/3
  Quaternions to Direction Cosine Matrix/1 -> Transpose/1
  Constant/1 -> MATLAB Function/3(dt)
  gyro/1 -> MATLAB Function/2(w)  "w"
  quat_0/1 -> Quaternions to Direction Cosine Matrix/1
  init_flag/1 -> Detect Increase/1

== system VB_RIFKF_GNSS_INS25/ISUS_RIEKF1/INS propogation/gyro bias compensation ==
  raw <gyro_B_rad/s_LPF> : Inport
  ddg : Inport  Port=2
  Measuemrnt Enable Flag : Inport  Port=3
  QGC_init : Inport  Port=4
  Add1 : Sum
  Data Type Conversion4 : DataTypeConversion  OutDataTypeStr=single  SaturateOnIntegerOverflow=off  RndMeth=Floor
  Scope1 : Scope
  error compensation : Subsystem
      settings: PortSchema="{\"entries\":[{\"content\":{\"sides\":[{\"content\":{\"connectorIds\":[\"In1\",\"In2\"]},\"type\":\"ConnectorPlacement.EquallySpacedRectSide\",\"uuid\":\"380e61a1-8124-48da-8c16-e78a4b6c30a9\"},{\"content\":{\"connectorIds\":[\"Out1\"],\"side\":\"RIGHT\"},\"type\":\"ConnectorPlacement.EquallySpacedRectSide\",\"uuid\":\"dacfd24e-67c3-4852-b5f7-795187362148\"},{\"content\":{\"side\":\"TOP\"},\"type\":\"ConnectorPlacement.EquallySpacedRectSide\",\"uuid\":\"56579dc4-3963-4476-a5d7-e0c30cfcd11c\"},{\"content\":{\"connectorIds\":[\"In3\"],\"side\":\"BOTTOM\"},\"type\":\"ConnectorPlacement.EquallySpacedRectSide\",\"uuid\":\"fc24e139-e918-40f2-99cc-0ca16c0a4a58\"}]},\"type\":\"ConnectorPlacement.EquallySpacedConnector\",\"uuid\":\"3ce5c04a-f8d2-476b-8ef1-0541292dfd95\"}],\"packageUris\":[\"http://schema.mathworks.com/mf0/Connector/R2020b\"],\"version\":\"1.0\"}"
  wb : Outport  PortDimensions=3
  dg : Outport  Port=2  PortDimensions=3
  wires:
  ddg/1 -> error compensation/1(ddg)
  QGC_init/1 -> error compensation/3(QGC_init)
  Add1/1 -> Data Type Conversion4/1
  Measuemrnt Enable Flag/1 -> error compensation/2(Enable)
  error compensation/1(dg) -> dg/1, Scope1/1, Add1/2
  raw <gyro_B_rad/s_LPF>/1 -> Add1/1
  Data Type Conversion4/1 -> wb/1

== system VB_RIFKF_GNSS_INS25/ISUS_RIEKF1/INS propogation/vel//pos update ==
  dtheta : Inport
  <DCM_b_n> : Inport  Port=2
  Ab : Inport  Port=3
  v0 : Inport  Port=4
  p0 : Inport  Port=5
  QGC_init : Inport  Port=6
  dp : Inport  Port=7
  dv : Inport  Port=8
  Kinematic Equation : Subsystem
  QGC_init1 : InportShadow  Port=6
  pos update : Subsystem
  vel update : Subsystem
  p_k : Outport  PortDimensions=3
  V : Outport  Port=2  PortDimensions=3
  wires:
  dtheta/1 -> vel update/1(dtheta), pos update/1(dtheta)
  vel update/1(vel_k) -> pos update/2(vel_k), V/1
  <DCM_b_n>/1 -> Kinematic Equation/1(Cbn)
  Ab/1 -> Kinematic Equation/2(Ab)
  QGC_init/1 -> vel update/2(QGC_init)
  Kinematic Equation/1(An) -> vel update/3(An)
  dv/1 -> vel update/4(KFState_dv)
  v0/1 -> vel update/5(v0)
  dp/1 -> pos update/3(dp)
  p0/1 -> pos update/5(p0)
  pos update/1(p_k) -> p_k/1
  QGC_init1/1 -> pos update/4(QGC_init)
